simulink model "dynamic_model_dab_range_test"  (R2022b)
settings: Solver=VariableStepAuto  StartTime=0.0  StopTime=100e-2  RelTol=1e-3
undefined symbols (not defined in the file): Ion, Lithium
libraries: spsSeriesRLCBranchLib x9, spsMosfetLib x8, spsMeanLib x6, eeGeneralControl x6, spsCurrentMeasurementLib x4, spsDiscreteVariableTimeDelayLib x2, spsEdgeDetectorLib x2, spsBatteryLib x1, spsDCVoltageSourceLib x1, spsMultimeterLib x1, spsStairGeneratorLib x1, slpidlib x1
settings Model: Creator=srikr  LastModifiedBy=srikri

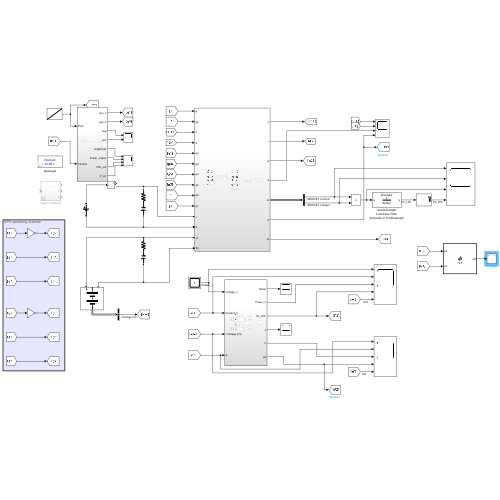
[thumbnail: Simulink's stored preview of the top-level diagram]
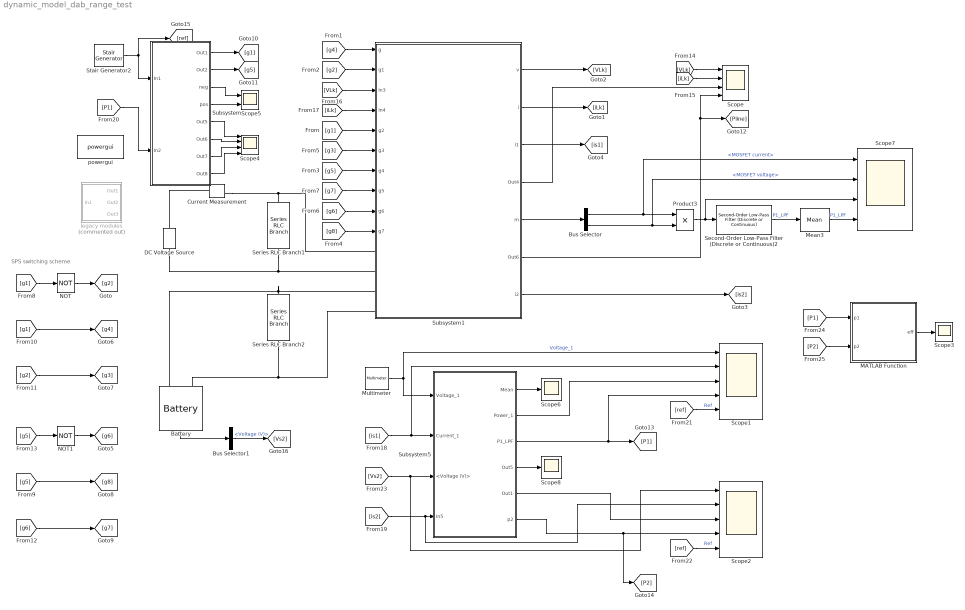
== system dynamic_model_dab_range_test ==
  note: SPS switching scheme
  Battery : spsBatteryLib/Battery  BatType=Lithium-Ion  ShowTempParam=off  ThermalPreset=no  ShowAgeParam=off  NomV=96  NomQ=150  SOC=100  Batt_Tr=30  PresetModel=on  MaxQ=150  MinV=72  FullV=111.7428  Dis_rate=65.2174  R=0.0064  Normal_OP=135.6522  expZone="[103.717      7.369565]"  current=[6.5 13 32.5]  Units=Time  Tci=20  NomT=20  T2=-30  MaxQ2=4.8  FullV2=7.1  Normal_OP2=5.655  expZone2="[6.58           1]"  Rca=0.6  ti=2000  Dp=0  Neq0=0  Tsim=1e6  Ta1=25  Qeol=5.4*0.9  Reol=0.013333*1.2  Char_age=[2.3478, 3]  Dis_age=[2.3478, 10]  N1=1500  N2=10500  N3=1000  N4=1400  Ta2=45  N5=950
  Bus Selector : BusSelector  OutputSignals=MOSFET current,MOSFET voltage
  Bus Selector1 : BusSelector  OutputSignals=Voltage (V)
  Current Measurement : spsCurrentMeasurementLib/Current Measurement  PhasorSimulation=off  OutputType=Complex  PSBequivalent=0
  DC Voltage Source : spsDCVoltageSourceLib/DC Voltage Source  Amplitude=120  Measurements=Voltage
  MATLAB Function : MATLAB Function  TreatAsAtomicUnit=on
  Mean3 : spsMeanLib/Mean  Freq=50e3  Vinit=0  Ts=0
  Multimeter : spsMultimeterLib/Multimeter  L=10  sel=4  yselected={}  Gain=1  OutputType=Complex  PlotAtSimulationStop=off  PhasorSimulation=off
  NOT : Logic  Operator=NOT  IconShape=distinctive  AllPortsSameDT=off  OutDataTypeStr=boolean
  NOT1 : Logic  Operator=NOT  IconShape=distinctive  AllPortsSameDT=off  OutDataTypeStr=boolean
  Product3 : Product
  Scope : Scope  NumInputPorts=4
  Scope1 : Scope  NumInputPorts=5
  Scope2 : Scope  NumInputPorts=5
  Scope3 : Scope
  Scope4 : Scope  NumInputPorts=4
  Scope5 : Scope  NumInputPorts=2
  Scope6 : Scope
  Scope7 : Scope  NumInputPorts=4
  Scope8 : Scope
  Second-Order Low-Pass Filter (Discrete or Continuous)2 : eeGeneralControl/Second-Order Low-Pass Filter (Discrete or Continuous)  A1=2*sqrt(2)*1e-3  A2=(1e-3)^2  init_option=Inherited from block input  x0=0  Ts=-1
      settings: LibrarySourceBlock=|
      | ee_sl_lib/General Control/Second-Order
      | Low-Pass Filter
      | (Discrete or Continuous)
  Series RLC Branch1 : spsSeriesRLCBranchLib/Series RLC Branch  LConnTagsString=__new0  RConnTagsString=__new0  BranchType=RC  Resistance=1e-9  Inductance=1e-3  SetiL0=off  InitialCurrent=0  Capacitance=1000e-6  Setx0=off  InitialVoltage=0  Measurements=None
  Series RLC Branch2 : spsSeriesRLCBranchLib/Series RLC Branch  LConnTagsString=__new0  RConnTagsString=__new0  BranchType=RC  Resistance=1e-9  Inductance=1e-3  SetiL0=off  InitialCurrent=0  Capacitance=1000e-6  Setx0=off  InitialVoltage=0  Measurements=None
  Stair Generator2 : spsStairGeneratorLib/Stair Generator  t=[0:0.025:1]*100e-2*(1-0.1)  e=([-1:0.05:1])*2.8e3  Ts=0
  Subsystem : Subsystem
  Subsystem1 : Subsystem
  Subsystem5 : Subsystem
  legacy modules : Subsystem  Commented=on
  powergui : spspowerguiLib/powergui  Priority=1  SimulationMode=Discrete  SampleTime=1e-6  frequency=60  Iterations=50  frequencyindice=0  Pbase=100e6  ErrMax=1e-4  UnitsV=kV  UnitsW=MW  buscounter=0  FunctionMessages=off  echomessages=off  EnableUseOfTLC=off  CurrentSourceSwitches=off  DisableSnubberDevices=off  DisableRonSwitches=off  DisableVfSwitches=off  DisplayEquations=off  AutomaticDiscreteSolvers=off  SolverType=Tustin/Backward Euler (TBE)  Interpol=off  ExternalGateDelay=off  methode=off  Ts=100  x0status=blocks  SPID=on  SwTol=0  HookPort=off  NonlinearTolerance=1e-4  nMaxIteration=100  ContinueOnMaxIteration=off  RestoreLinks=warning  ResistiveCurrentMeasurement=off  Frange=[0:2:500]  Ylog=off  Xlog=on  ShowGrid=off  save=off  variable=ZData  structure=0  ZoomFFT=off  StartTime=0.0  cycles=1  DisplayStyle=1  fundamental=60  FreqAxis=off  MaxFrequency=1000  frequencyindicesteady=1  RmsSteady=1  display=off
  wires:
  [VLk] -> Scope/1
  [iLk] -> Scope/2
  Multimeter/1 -> Scope1/1, Subsystem5/1(Voltage_1)  "Voltage_1"
  [is2] -> Scope2/2, Subsystem5/4(In5)
  Stair Generator2/1 -> Subsystem/1(In1), [ref]
  Bus Selector/1 -> Scope7/1, Product3/1  "<MOSFET current>"
  Bus Selector/2 -> Scope7/2, Product3/2  "<MOSFET voltage>"
  Product3/1 -> Scope7/3, Second-Order Low-Pass Filter (Discrete or Continuous)2/1
  [ref] -> Scope1/5  "Ref"
  Battery/1 -> Bus Selector1/1
  [P1] -> Subsystem/2(In2)
  Subsystem/1(Out1) -> [g1]
  Subsystem/2(Out2) -> [g5]
  Subsystem/3(neg) -> Scope5/1
  Subsystem/4(pos) -> Scope5/2
  Subsystem/5(Out5) -> Scope4/1
  Subsystem/6(Out6) -> Scope4/2
  Subsystem/7(Out7) -> Scope4/3
  Subsystem/8(Out8) -> Scope4/4
  Subsystem5/1(Mean) -> Scope6/1
  Subsystem5/2(Power_1) -> Scope1/3
  Subsystem1/6(Out6) -> [Pline], Scope/4
  [g4] -> Subsystem1/1(g)
  [g2] -> Subsystem1/2(g1)
  [VLk] -> Subsystem1/3(In3)
  [iLk] -> Subsystem1/4(In4)
  [g1] -> Subsystem1/5(g2)
  [g3] -> Subsystem1/6(g3)
  [g5] -> Subsystem1/7(g4)
  [g7] -> Subsystem1/8(g5)
  [g6] -> Subsystem1/9(g6)
  [g8] -> Subsystem1/10(g7)
  Subsystem1/1(v) -> [VLk]
  Subsystem1/2(i) -> [iLk]
  Subsystem1/3(i1) -> [is1]
  Subsystem1/4(Out4) -> Scope/3
  Subsystem1/5(m) -> Bus Selector/1
  Subsystem1/7(i2) -> [is2]
  [g1] -> NOT/1
  NOT/1 -> [g2]
  [g5] -> [g8]
  NOT1/1 -> [g6]
  [g6] -> [g7]
  [g5] -> NOT1/1
  [g2] -> [g3]
  [g1] -> [g4]
  Subsystem5/5(Out1) -> Scope2/3
  [is1] -> Scope1/2, Subsystem5/2(Current_1)
  [ref] -> Scope2/5  "Ref"
  Bus Selector1/1 -> [Vs2]  "<Voltage (V)>"
  [Vs2] -> Scope2/1, Subsystem5/3(<Voltage (V)>)
  Second-Order Low-Pass Filter (Discrete or Continuous)2/1 -> Mean3/1  "P1_LPF"
  Mean3/1 -> Scope7/4  "P1_LPF"
  Subsystem5/3(P1_LPF) -> [P1], Scope1/4
  MATLAB Function/1(eff) -> Scope3/1
  Subsystem5/4(Out5) -> Scope8/1
  Subsystem5/6(p2) -> [P2], Scope2/4
  [P1] -> MATLAB Function/1(p1)
  [P2] -> MATLAB Function/2(p2)
  connections:
  Series RLC Branch1/RConn1 -- DC Voltage Source/LConn1 -- Subsystem1/LConn2
  Series RLC Branch2/RConn1 -- Battery/LConn2 -- Subsystem1/LConn4
  Series RLC Branch2/LConn1 -- Battery/LConn1 -- Subsystem1/LConn3
  Subsystem1/LConn1 -- Current Measurement/RConn1 -- Series RLC Branch1/LConn1
  Current Measurement/LConn1 -- DC Voltage Source/RConn1

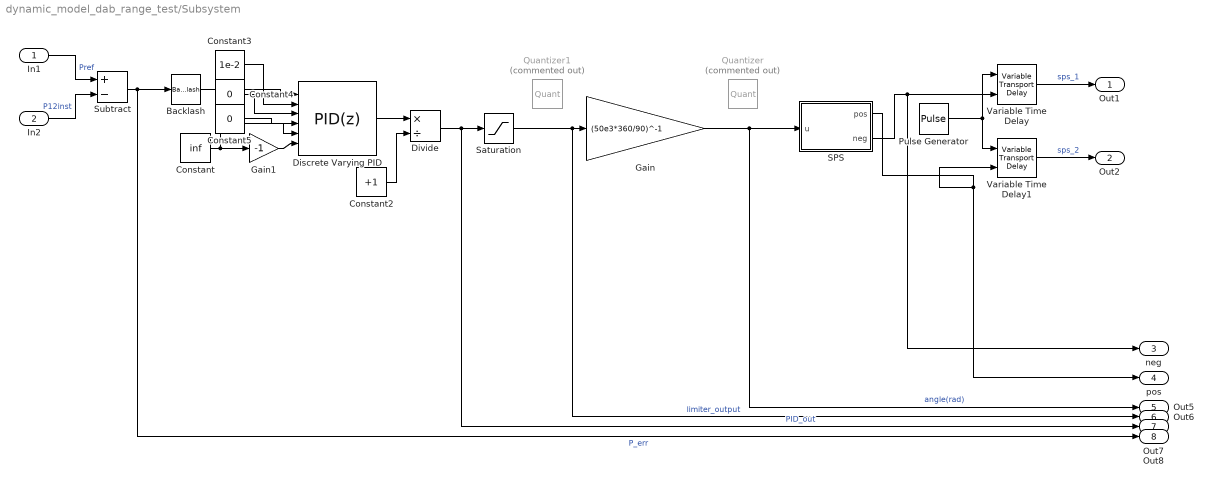
== system dynamic_model_dab_range_test/Subsystem ==
  In1 : Inport
  In2 : Inport  Port=2
  Backlash : Backlash  BacklashWidth=0
  Constant : Constant  Value=inf
  Constant2 : Constant  Value=+1
  Constant3 : Constant  Value=1e-2
  Constant4 : Constant  Value=0
  Constant5 : Constant  Value=0
  Discrete Varying PID : slpidlib/PID Controller  Controller=PID  Form=Parallel  TimeDomain=Discrete-time  UseExternalTs=off  SampleTime=-1  IntegratorMethod=Forward Euler  FilterMethod=Forward Euler  ControllerParametersSource=external  P=1  I=1  UseKiTs=off  D=0  N=100  UseFilter=off  TunerSelectOption=Transfer Function Based (PID Tuner App)  InitialConditionSource=internal  InitialConditionForIntegrator=0  InitialConditionForFilter=0  DifferentiatorICPrevScaledInput=0  ExternalReset=none  TrackingMode=off  Kt=1  LimitOutput=on  SatLimitsSource=external  UpperSaturationLimit=inf  LowerSaturationLimit=-inf  LinearizeAsGain=on  AntiWindupMode=none  Kb=1  LimitIntegrator=off  UpperIntegratorSaturationLimit=inf  LowerIntegratorSaturationLimit=-inf  POutMin=[]  POutMax=[]  IOutMin=[]  IOutMax=[]  DOutMin=[]  DOutMax=[]  NOutMin=[]  NOutMax=[]  SumOutMin=[]  SumOutMax=[]  SaturationOutMin=[]  SaturationOutMax=[]  PParamMin=[]  PParamMax=[]  IParamMin=[]  IParamMax=[]  DParamMin=[]  DParamMax=[]  NParamMin=[]  NParamMax=[]  KbParamMin=[]  KbParamMax=[]  KtParamMin=[]  KtParamMax=[]  KbOutMin=[]  KbOutMax=[]  KtOutMin=[]  KtOutMax=[]  IntegratorOutMin=[]  IntegratorOutMax=[]  FilterOutMin=[]  FilterOutMax=[]  SumI1OutMin=[]  SumI1OutMax=[]  SumI2OutMin=[]  SumI2OutMax=[]  SumI3OutMin=[]  SumI3OutMax=[]  SumI4OutMin=[]  SumI4OutMax=[]  SumDOutMin=[]  SumDOutMax=[]  DifferentiatorOutMin=[]  DifferentiatorOutMax=[]  FilterDiffOutCoefMin=[]  FilterDiffOutCoefMax=[]  ReciprocalOutMin=[]  ReciprocalOutMax=[]  SumDenOutMin=[]  SumDenOutMax=[]  SumNumOutMin=[]  SumNumOutMax=[]  DivideOutMin=[]  DivideOutMax=[]  UdiffTsProdOutMin=[]  UdiffTsProdOutMax=[]  NTsProdOutMin=[]  NTsProdOutMax=[]  UintegralTsProdOutMin=[]  UintegralTsProdOutMax=[]  UngainTsProdOutMin=[]  UngainTsProdOutMax=[]  ClampingZeroOutDataTypeStr=Inherit: Inherit via back propagation  ClampingZeroOutMin=[]  ClampingZeroOutMax=[]  FilterDenConstantOutDataTypeStr=Inherit: Inherit via back propagation  FilterDenConstantOutMin=[]  FilterDenConstantOutMax=[]  PCopyOutDataTypeStr=Inherit: Inherit via back propagation  PCopyOutMin=[]  PCopyOutMax=[]  NCopyOutDataTypeStr=Inherit: Inherit via back propagation  NCopyOutMin=[]  NCopyOutMax=[]  IntegratorContinuousStateAttributes=''  IntegratorStateMustResolveToSignalObject=off  IntegratorRTWStateStorageClass=Auto  FilterContinuousStateAttributes=''  FilterStateMustResolveToSignalObject=off  FilterRTWStateStorageClass=Auto  ParallelPVariant=ExternalParameters  IdealPVariant=Disabled  IVariant=ExternalParameters  DVariant=ExternalParameters  IntegratorVariant=Discrete  SatVariant=External  AWVariant=Passthrough  PCopyVariant=Disabled  TRVariant=Disabled  FdbkBlocksVariant=Forward  IdealPFdbkVariant=Disabled  SatFdbkVariant=Disabled  DerivativeFilterVariant=Differentiator  NVariant=Passthrough  NCopyVariant=Disabled_SignalSpec  FilterICVariant=InternalICsDifferentiator  IntegratorICVariant=InternalICs  ExternalResetVariant=Disabled  TRSumVariant=Passthrough  SumFdbkVariant=Disabled  SumVariant=Sum_PID  TsampFilterVariant=InternalTs  TsampNgainVariant=Passthrough  TsampIntegralVariant=Passthrough  ExternalSaturationOutDataTypeStr=Inherit: Same as second input
      settings: LibrarySourceBlock=cstblocks/Linear Parameter Varying/Discrete Varying PID
  Divide : Product  Inputs=*/
  Gain : Gain  Gain=(50e3*360/90)^-1
  Gain1 : Gain  Gain=-1
  Pulse Generator : DiscretePulseGenerator  PulseType=Time based  Period=1/50e3  PulseWidth=50
  Quantizer : Quantizer  Commented=on  QuantizationInterval=1e-5
  Quantizer1 : Quantizer  Commented=on  QuantizationInterval=1e-2
  SPS : MATLAB Function  TreatAsAtomicUnit=on
  Saturation : Saturate  UpperLimit=1  LowerLimit=-1
  Subtract : Sum  Inputs=+-
  Variable Time Delay : VariableTransportDelay  MaximumDelay=10
  Variable Time Delay1 : VariableTransportDelay  MaximumDelay=10
  Out1 : Outport
  Out2 : Outport  Port=2
  neg : Outport  Port=3
  pos : Outport  Port=4
  Out5 : Outport  Port=5
  Out6 : Outport  Port=6
  Out7 : Outport  Port=7
  Out8 : Outport  Port=8
  wires:
  Backlash/1 -> Discrete Varying PID/1
  Constant2/1 -> Divide/2
  Constant4/1 -> Discrete Varying PID/3
  In1/1 -> Subtract/1  "Pref"
  Variable Time Delay/1 -> Out1/1  "sps_1"
  Saturation/1 -> Out6/1, Gain/1  "limiter_output"
  SPS/1(pos) -> pos/1, Variable Time Delay1/2
  SPS/2(neg) -> neg/1, Variable Time Delay/2
  Variable Time Delay1/1 -> Out2/1  "sps_2"
  In2/1 -> Subtract/2  "P12inst"
  Constant/1 -> Discrete Varying PID/5, Gain1/1
  Constant5/1 -> Discrete Varying PID/4
  Pulse Generator/1 -> Variable Time Delay1/1, Variable Time Delay/1
  Constant3/1 -> Discrete Varying PID/2
  Divide/1 -> Out7/1, Saturation/1  "PID_out"
  Discrete Varying PID/1 -> Divide/1
  Subtract/1 -> Out8/1, Backlash/1  "P_err"
  Gain1/1 -> Discrete Varying PID/6
  Gain/1 -> Out5/1, SPS/1(u)  "angle(rad)"

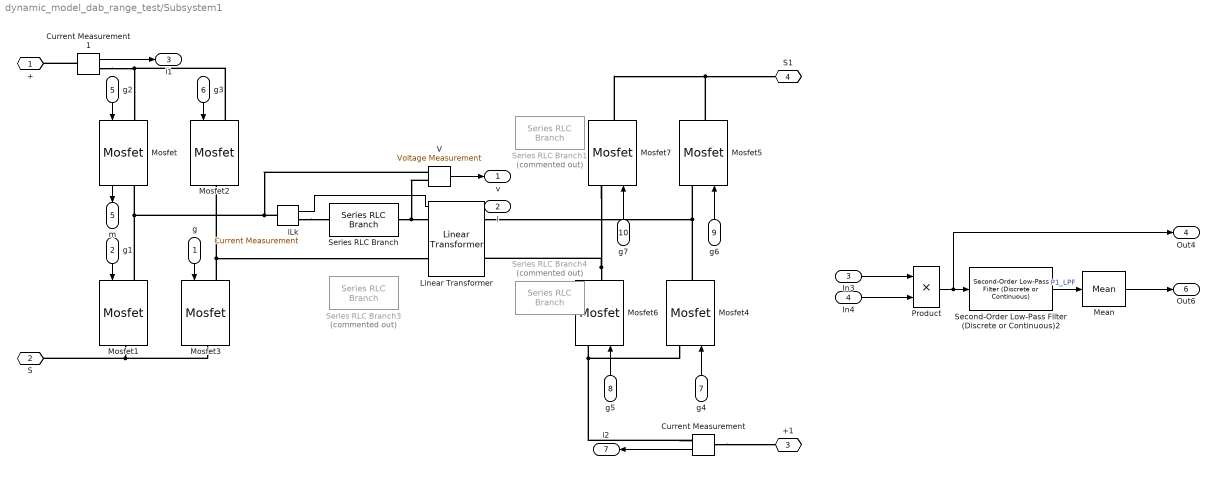
== system dynamic_model_dab_range_test/Subsystem1 ==
  g : Inport
  g1 : Inport  Port=2
  In3 : Inport  Port=3
  In4 : Inport  Port=4
  g2 : Inport  Port=5
  g3 : Inport  Port=6
  g4 : Inport  Port=7
  g5 : Inport  Port=8
  g6 : Inport  Port=9
  g7 : Inport  Port=10
  Current Measurement : spsCurrentMeasurementLib/Current Measurement  PhasorSimulation=off  OutputType=Complex  PSBequivalent=0
  Current Measurement1 : spsCurrentMeasurementLib/Current Measurement  PhasorSimulation=off  OutputType=Complex  PSBequivalent=0
  Linear Transformer : spsLinearTransformerLib/Linear Transformer  UNITS=SI  NominalPower=[ 3.5e3 50e3 ]  winding1=[120 0 0]  winding2=[96 0 0]  ThreeWindings=off  winding3=[3.15e+05 0.7938 0.084225]  RmLm=[10e6 2e-3]  Measurements=All voltages and currents  DataType=on
  Mean : spsMeanLib/Mean  Freq=50e3  Vinit=0  Ts=0
  Mosfet : spsMosfetLib/Mosfet  Ron=0.1  Lon=0  Rd=0.01  Vfd=0  IC=0  Rs=1e6  Cs=inf  Measurements=on
  Mosfet1 : spsMosfetLib/Mosfet  Ron=0.1  Lon=0  Rd=0.01  Vfd=0  IC=0  Rs=inf  Cs=inf  Measurements=off
  Mosfet{2..7} (6 alike) : spsMosfetLib/Mosfet  Ron=0.1  Lon=0  Rd=0.01  Vfd=0  IC=0  Rs=1e6  Cs=inf  Measurements=off
  Product : Product
  Second-Order Low-Pass Filter (Discrete or Continuous)2 : eeGeneralControl/Second-Order Low-Pass Filter (Discrete or Continuous)  A1=2*sqrt(2)*1e-3  A2=(1e-3)^2  init_option=Inherited from block input  x0=0  Ts=-1
      settings: LibrarySourceBlock=|
      | ee_sl_lib/General Control/Second-Order
      | Low-Pass Filter
      | (Discrete or Continuous)
  Series RLC Branch : spsSeriesRLCBranchLib/Series RLC Branch  LConnTagsString=__new0  RConnTagsString=__new0  BranchType=L  Resistance=1  Inductance=14e-6  SetiL0=off  InitialCurrent=0  Capacitance=1e-6  Setx0=off  InitialVoltage=0  Measurements=Branch voltage and current
  Series RLC Branch1 : spsSeriesRLCBranchLib/Series RLC Branch  Commented=on  LConnTagsString=__new0  RConnTagsString=__new0  BranchType=L  Resistance=1  Inductance=80e-6  SetiL0=off  InitialCurrent=0  Capacitance=1e-6  Setx0=off  InitialVoltage=0  Measurements=Branch voltage and current
  Series RLC Branch3 : spsSeriesRLCBranchLib/Series RLC Branch  Commented=on  LConnTagsString=__new0  RConnTagsString=__new0  BranchType=C  Resistance=1  Inductance=15e-6  SetiL0=off  InitialCurrent=0  Capacitance=0.127e-6  Setx0=off  InitialVoltage=0  Measurements=Branch voltage and current
  Series RLC Branch4 : spsSeriesRLCBranchLib/Series RLC Branch  Commented=on  LConnTagsString=__new0  RConnTagsString=__new0  BranchType=C  Resistance=1  Inductance=15e-6  SetiL0=off  InitialCurrent=0  Capacitance=0.127e-6  Setx0=off  InitialVoltage=0  Measurements=Branch voltage and current
  V : spsVoltageMeasurementLib/Voltage Measurement  PhasorSimulation=off  OutputType=Complex  PSBequivalent=0
  iLk : spsCurrentMeasurementLib/Current Measurement  PhasorSimulation=off  OutputType=Complex  PSBequivalent=0
  + : PMIOPort  Side=Left
  S : PMIOPort  Port=2  Side=Left
  +1 : PMIOPort  Port=3  Side=Left
  S1 : PMIOPort  Port=4  Side=Left
  v : Outport
  i : Outport  Port=2
  i1 : Outport  Port=3
  Out4 : Outport  Port=4
  m : Outport  Port=5
  Out6 : Outport  Port=6
  i2 : Outport  Port=7
  wires:
  V/1 -> v/1
  g5/1 -> Mosfet6/1
  In3/1 -> Product/1
  g6/1 -> Mosfet5/1
  In4/1 -> Product/2
  Mosfet/1 -> m/1
  g2/1 -> Mosfet/1
  g4/1 -> Mosfet4/1
  iLk/1 -> i/1
  Current Measurement1/1 -> i1/1
  Current Measurement/1 -> i2/1
  g1/1 -> Mosfet1/1
  g/1 -> Mosfet3/1
  Mean/1 -> Out6/1
  g3/1 -> Mosfet2/1
  g7/1 -> Mosfet7/1
  Product/1 -> Out4/1, Second-Order Low-Pass Filter (Discrete or Continuous)2/1
  Second-Order Low-Pass Filter (Discrete or Continuous)2/1 -> Mean/1  "P1_LPF"
  connections:
  Current Measurement1/RConn1 -- Mosfet/LConn1 -- Mosfet2/LConn1
  Series RLC Branch/RConn1 -- V/LConn2 -- Linear Transformer/LConn1
  Current Measurement/LConn1 -- +1/RConn1
  Current Measurement/RConn1 -- Mosfet4/LConn1 -- Mosfet6/LConn1
  Current Measurement1/LConn1 -- +/RConn1
  Mosfet3/RConn1 -- S/RConn1 -- Mosfet1/RConn1
  iLk/LConn1 -- V/LConn1 -- Mosfet/RConn1 -- Mosfet1/LConn1
  iLk/RConn1 -- Series RLC Branch/LConn1
  Mosfet7/RConn1 -- Mosfet5/RConn1 -- S1/RConn1
  Mosfet3/LConn1 -- Linear Transformer/LConn2 -- Mosfet2/RConn1
  Mosfet4/RConn1 -- Mosfet5/LConn1 -- Linear Transformer/RConn1
  Mosfet6/RConn1 -- Linear Transformer/RConn2 -- Mosfet7/LConn1

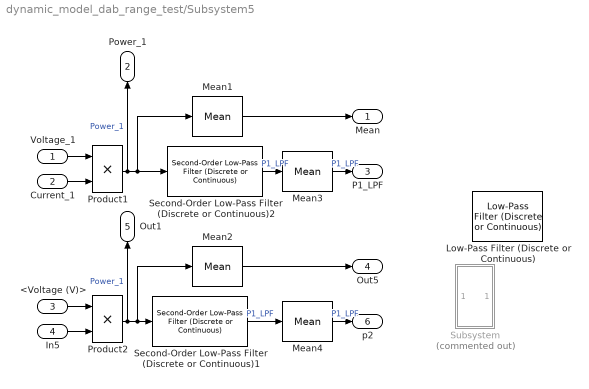
== system dynamic_model_dab_range_test/Subsystem5 ==
  Voltage_1 : Inport
  Current_1 : Inport  Port=2
  <Voltage (V)> : Inport  Port=3
  In5 : Inport  Port=4
  Low-Pass Filter (Discrete or Continuous) : eeGeneralControl/Low-Pass Filter (Discrete or Continuous)  K=1  T=1e-3  B=inf  A=-inf  init_option=Specify as parameter  x0=0  Ts=-1
  Mean{1..4} (4 alike) : spsMeanLib/Mean  Freq=50e3  Vinit=0  Ts=0
  Product1 : Product
  Product2 : Product
  Second-Order Low-Pass Filter (Discrete or Continuous)1 : eeGeneralControl/Second-Order Low-Pass Filter (Discrete or Continuous)  A1=1e-3  A2=1e-6  init_option=Inherited from block input  x0=0  Ts=-1
      settings: LibrarySourceBlock=|
      | ee_sl_lib/General Control/Second-Order
      | Low-Pass Filter
      | (Discrete or Continuous)
  Second-Order Low-Pass Filter (Discrete or Continuous)2 : eeGeneralControl/Second-Order Low-Pass Filter (Discrete or Continuous)  A1=2*sqrt(2)*1e-3  A2=(1e-3)^2  init_option=Inherited from block input  x0=0  Ts=-1
      settings: LibrarySourceBlock=|
      | ee_sl_lib/General Control/Second-Order
      | Low-Pass Filter
      | (Discrete or Continuous)
  Subsystem : Subsystem  Commented=on
  Mean : Outport
  Power_1 : Outport  Port=2
  P1_LPF : Outport  Port=3
  Out5 : Outport  Port=4
  Out1 : Outport  Port=5
  p2 : Outport  Port=6
  wires:
  Current_1/1 -> Product1/2
  Mean1/1 -> Mean/1
  Product1/1 -> Mean1/1, Second-Order Low-Pass Filter (Discrete or Continuous)2/1, Power_1/1  "Power_1"
  <Voltage (V)>/1 -> Product2/1
  Voltage_1/1 -> Product1/1
  In5/1 -> Product2/2
  Mean2/1 -> Out5/1
  Mean3/1 -> P1_LPF/1  "P1_LPF"
  Second-Order Low-Pass Filter (Discrete or Continuous)1/1 -> Mean4/1  "P1_LPF"
  Product2/1 -> Mean2/1, Second-Order Low-Pass Filter (Discrete or Continuous)1/1, Out1/1  "Power_1"
  Mean4/1 -> p2/1  "P1_LPF"
  Second-Order Low-Pass Filter (Discrete or Continuous)2/1 -> Mean3/1  "P1_LPF"

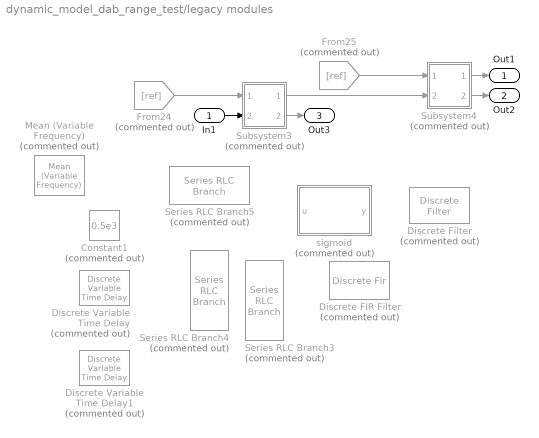
== system dynamic_model_dab_range_test/legacy modules ==
  In1 : Inport
  Constant1 : Constant  Commented=on  Value=0.5e3
  Discrete FIR Filter : DiscreteFir  Commented=on
  Discrete Filter : DiscreteFilter  Commented=on
  Discrete Variable Time Delay : spsDiscreteVariableTimeDelayLib/Discrete Variable Time Delay  Commented=on  MaxDelay=1  InitialValue=0  Ts=1e-4  DFT=on
      settings: LibrarySourceBlock=|
      | sps_lib/Control/Discrete Variable
      | Time Delay
  Discrete Variable Time Delay1 : spsDiscreteVariableTimeDelayLib/Discrete Variable Time Delay  Commented=on  MaxDelay=1  InitialValue=0  Ts=1e-4  DFT=on
      settings: LibrarySourceBlock=|
      | sps_lib/Control/Discrete Variable
      | Time Delay
  From24 : From  Commented=on  GotoTag=ref
  From25 : From  Commented=on  GotoTag=ref
  Mean (Variable Frequency) : spsMeanVariableFrequencyLib/Mean (Variable Frequency)  Commented=on  Finit=60  Fmin=45  Vinit=0  Ts=0
      settings: LibrarySourceBlock=|
      | sps_lib/Sensors and Measurements/Mean
      | (Variable Frequency)
  Series RLC Branch3 : spsSeriesRLCBranchLib/Series RLC Branch  Commented=on  LConnTagsString=__new0  RConnTagsString=__new0  BranchType=L  Resistance=1  Inductance=1e-6/(1.25^2)  SetiL0=off  InitialCurrent=0  Capacitance=1e-6  Setx0=off  InitialVoltage=0  Measurements=Branch voltage and current
  Series RLC Branch4 : spsSeriesRLCBranchLib/Series RLC Branch  Commented=on  LConnTagsString=__new0  RConnTagsString=__new0  BranchType=C  Resistance=1  Inductance=14e-6  SetiL0=off  InitialCurrent=0  Capacitance=10e-6*(1.25^2)  Setx0=off  InitialVoltage=0  Measurements=Branch voltage and current
  Series RLC Branch5 : spsSeriesRLCBranchLib/Series RLC Branch  Commented=on  LConnTagsString=__new0  RConnTagsString=__new0  BranchType=C  Resistance=1  Inductance=14e-6  SetiL0=off  InitialCurrent=0  Capacitance=10e-6  Setx0=off  InitialVoltage=0  Measurements=Branch voltage and current
  Subsystem3 : Subsystem  Commented=on
  Subsystem4 : Subsystem  Commented=on
  sigmoid : MATLAB Function  Commented=on  TreatAsAtomicUnit=on
  Out1 : Outport
  Out2 : Outport  Port=2
  Out3 : Outport  Port=3
  wires:
  Subsystem3/1(Out1) -> Subsystem4/2(In2)
  From25/1 -> Subsystem4/1(In1)
  From24/1 -> Subsystem3/1(In1)
  In1/1 -> Subsystem3/2(In2)
  Subsystem4/2(Out2) -> Out2/1
  Subsystem4/1(Out1) -> Out1/1
  Subsystem3/2(Out2) -> Out3/1

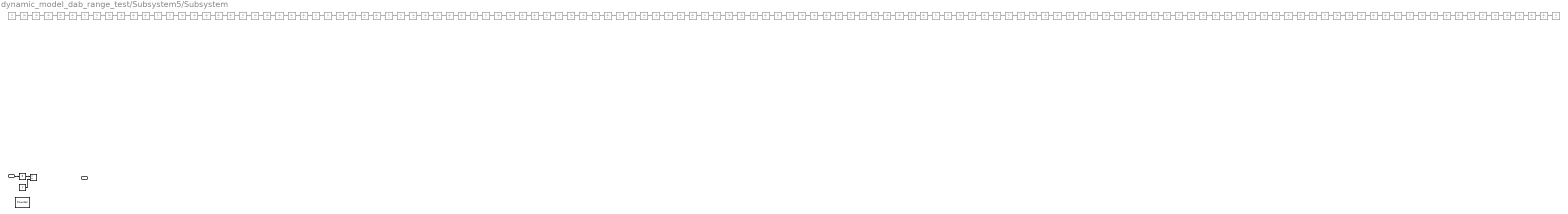
== system dynamic_model_dab_range_test/Subsystem5/Subsystem ==
  In1 : Inport
  Constant : Constant
  Counter : eeGeneralControl/Counter  CarrCount=Up  Range=[0 1]  Tper=0.001  Tdelay=0  Ts=0.0001
      settings: LibrarySourceBlock=ee_sl_lib/General Control/Counter
  Divide : Product  Inputs=*/
  Sum of Elements : Sum  Inputs=+  AccumDataTypeStr=int16  SaturateOnIntegerOverflow=on
  Unit Delay{,1..127} (128 alike) : UnitDelay  Commented=on  SampleTime=-1  HasFrameUpgradeWarning=on
  Out1 : Outport
  wires:
  In1/1 -> Sum of Elements/1
  Unit Delay65/1 -> Unit Delay120/1
  Unit Delay126/1 -> Unit Delay127/1
  Unit Delay2/1 -> Unit Delay3/1
  Unit Delay64/1 -> Unit Delay65/1
  Unit Delay125/1 -> Unit Delay98/1
  Unit Delay/1 -> Unit Delay1/1
  Unit Delay82/1 -> Unit Delay72/1
  Unit Delay75/1 -> Unit Delay88/1
  Unit Delay88/1 -> Unit Delay89/1
  Unit Delay72/1 -> Unit Delay73/1
  Unit Delay86/1 -> Unit Delay83/1
  Unit Delay40/1 -> Unit Delay41/1
  Unit Delay17/1 -> Unit Delay28/1
  Unit Delay69/1 -> Unit Delay81/1
  Unit Delay116/1 -> Unit Delay117/1
  Unit Delay87/1 -> Unit Delay64/1
  Unit Delay10/1 -> Unit Delay11/1
  Unit Delay96/1 -> Unit Delay97/1
  Unit Delay78/1 -> Unit Delay103/1
  Unit Delay115/1 -> Unit Delay90/1
  Unit Delay46/1 -> Unit Delay76/1
  Unit Delay77/1 -> Unit Delay78/1
  Unit Delay90/1 -> Unit Delay91/1
  Unit Delay98/1 -> Unit Delay109/1
  Unit Delay26/1 -> Unit Delay27/1
  Unit Delay100/1 -> Unit Delay113/1
  Unit Delay68/1 -> Unit Delay69/1
  Unit Delay120/1 -> Unit Delay125/1
  Unit Delay12/1 -> Unit Delay13/1
  Unit Delay112/1 -> Unit Delay101/1
  Unit Delay50/1 -> Unit Delay40/1
  Unit Delay103/1 -> Unit Delay115/1
  Unit Delay80/1 -> Unit Delay77/1
  Unit Delay124/1 -> Unit Delay96/1
  Unit Delay38/1 -> Unit Delay39/1
  Unit Delay84/1 -> Unit Delay74/1
  Unit Delay73/1 -> Unit Delay85/1
  Unit Delay56/1 -> Unit Delay57/1
  Unit Delay118/1 -> Unit Delay119/1
  Unit Delay89/1 -> Unit Delay79/1
  Unit Delay44/1 -> Unit Delay55/1
  Unit Delay94/1 -> Unit Delay95/1
  Unit Delay43/1 -> Unit Delay56/1
  Unit Delay81/1 -> Unit Delay82/1
  Unit Delay79/1 -> Unit Delay80/1
  Unit Delay58/1 -> Unit Delay59/1
  Unit Delay24/1 -> Unit Delay25/1
  Unit Delay85/1 -> Unit Delay86/1
  Unit Delay97/1 -> Unit Delay94/1
  Unit Delay104/1 -> Unit Delay105/1
  Unit Delay71/1 -> Unit Delay68/1
  Unit Delay127/1 -> Unit Delay70/1
  Unit Delay76/1 -> Unit Delay87/1
  Unit Delay7/1 -> Unit Delay4/1
  Unit Delay108/1 -> Unit Delay110/1
  Unit Delay110/1 -> Unit Delay99/1
  Unit Delay107/1 -> Unit Delay104/1
  Unit Delay117/1 -> Unit Delay106/1
  Unit Delay54/1 -> Unit Delay51/1
  Unit Delay61/1 -> Unit Delay58/1
  Unit Delay122/1 -> Unit Delay118/1
  Unit Delay93/1 -> Unit Delay123/1
  Unit Delay59/1 -> Unit Delay34/1
  Unit Delay51/1 -> Unit Delay52/1
  Unit Delay114/1 -> Unit Delay111/1
  Unit Delay95/1 -> Unit Delay108/1
  Unit Delay83/1 -> Unit Delay84/1
  Unit Delay106/1 -> Unit Delay107/1
  Unit Delay13/1 -> Unit Delay24/1
  Unit Delay113/1 -> Unit Delay114/1
  Unit Delay91/1 -> Unit Delay121/1
  Unit Delay25/1 -> Unit Delay16/1
  Unit Delay121/1 -> Unit Delay122/1
  Unit Delay66/1 -> Unit Delay67/1
  Unit Delay29/1 -> Unit Delay26/1
  Unit Delay101/1 -> Unit Delay102/1
  Unit Delay111/1 -> Unit Delay112/1
  Unit Delay30/1 -> Unit Delay31/1
  Unit Delay70/1 -> Unit Delay71/1
  Unit Delay119/1 -> Unit Delay92/1
  Unit Delay18/1 -> Unit Delay19/1
  Unit Delay67/1 -> Unit Delay126/1
  Unit Delay74/1 -> Unit Delay75/1
  Unit Delay28/1 -> Unit Delay29/1
  Unit Delay102/1 -> Unit Delay116/1
  Unit Delay6/1 -> Unit Delay7/1
  Unit Delay31/1 -> Unit Delay22/1
  Unit Delay63/1 -> Unit Delay38/1
  Unit Delay16/1 -> Unit Delay17/1
  Unit Delay19/1 -> Unit Delay30/1
  Unit Delay22/1 -> Unit Delay23/1
  Unit Delay20/1 -> Unit Delay21/1
  Unit Delay62/1 -> Unit Delay63/1
  Unit Delay32/1 -> Unit Delay33/1
  Unit Delay39/1 -> Unit Delay36/1
  Unit Delay35/1 -> Unit Delay62/1
  Unit Delay37/1 -> Unit Delay49/1
  Unit Delay33/1 -> Unit Delay60/1
  Unit Delay3/1 -> Unit Delay/1
  Unit Delay21/1 -> Unit Delay44/1
  Unit Delay47/1 -> Unit Delay48/1
  Unit Delay42/1 -> Unit Delay43/1
  Unit Delay60/1 -> Unit Delay61/1
  Unit Delay41/1 -> Unit Delay53/1
  Unit Delay23/1 -> Unit Delay20/1
  Unit Delay55/1 -> Unit Delay32/1
  Unit Delay34/1 -> Unit Delay35/1
  Unit Delay11/1 -> Unit Delay8/1
  Unit Delay15/1 -> Unit Delay12/1
  Unit Delay14/1 -> Unit Delay15/1
  Unit Delay53/1 -> Unit Delay54/1
  Unit Delay99/1 -> Unit Delay100/1
  Unit Delay49/1 -> Unit Delay50/1
  Unit Delay45/1 -> Unit Delay46/1
  Unit Delay9/1 -> Unit Delay14/1
  Unit Delay36/1 -> Unit Delay37/1
  Unit Delay123/1 -> Unit Delay124/1
  Unit Delay109/1 -> Unit Delay66/1
  Unit Delay92/1 -> Unit Delay93/1
  Unit Delay5/1 -> Unit Delay10/1
  Unit Delay48/1 -> Unit Delay45/1
  Unit Delay57/1 -> Unit Delay47/1
  Unit Delay52/1 -> Unit Delay42/1
  Unit Delay27/1 -> Unit Delay18/1
  Unit Delay4/1 -> Unit Delay5/1
  Unit Delay8/1 -> Unit Delay9/1
  Unit Delay1/1 -> Unit Delay6/1
  Sum of Elements/1 -> Divide/1
  Constant/1 -> Divide/2

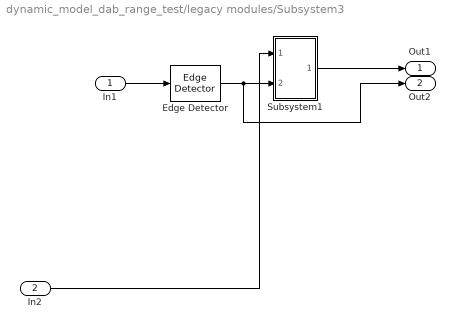
== system dynamic_model_dab_range_test/legacy modules/Subsystem3 ==
  In1 : Inport
  In2 : Inport  Port=2
  Edge Detector : spsEdgeDetectorLib/Edge Detector  model=Either  ic=0  Ts=0
      settings: LibrarySourceBlock=sps_lib/Control/Edge Detector
  Subsystem1 : Subsystem
  Out1 : Outport
  Out2 : Outport  Port=2
  wires:
  Edge Detector/1 -> Out2/1, Subsystem1/2(Input)
  Subsystem1/1(Out1) -> Out1/1
  In1/1 -> Edge Detector/1
  In2/1 -> Subsystem1/1(In1)

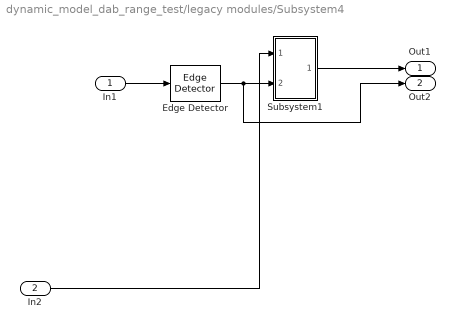
== system dynamic_model_dab_range_test/legacy modules/Subsystem4 ==
  In1 : Inport
  In2 : Inport  Port=2
  Edge Detector : spsEdgeDetectorLib/Edge Detector  model=Either  ic=0  Ts=0
      settings: LibrarySourceBlock=sps_lib/Control/Edge Detector
  Subsystem1 : Subsystem
  Out1 : Outport
  Out2 : Outport  Port=2
  wires:
  Edge Detector/1 -> Out2/1, Subsystem1/2(Input)
  Subsystem1/1(Out1) -> Out1/1
  In1/1 -> Edge Detector/1
  In2/1 -> Subsystem1/1(In1)

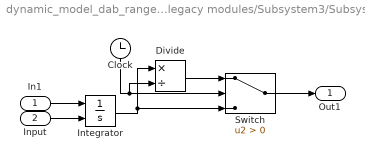
== system dynamic_model_dab_range_test/legacy modules/Subsystem3/Subsystem1 ==
  In1 : Inport
  Input : Inport  Port=2
  Clock : Clock
  Divide : Product  Inputs=*/
  Integrator : Integrator  ExternalReset=rising  LimitOutput=on  IgnoreLimit=on
  Switch : Switch  Criteria=u2 > Threshold  SaturateOnIntegerOverflow=off  InputSameDT=off
  Out1 : Outport
  wires:
  Divide/1 -> Switch/1
  Integrator/1 -> Switch/3, Divide/1
  Clock/1 -> Switch/2, Divide/2
  In1/1 -> Integrator/1
  Switch/1 -> Out1/1
  Input/1 -> Integrator/2

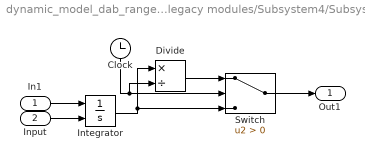
== system dynamic_model_dab_range_test/legacy modules/Subsystem4/Subsystem1 ==
  In1 : Inport
  Input : Inport  Port=2
  Clock : Clock
  Divide : Product  Inputs=*/
  Integrator : Integrator  ExternalReset=rising  LimitOutput=on  IgnoreLimit=on
  Switch : Switch  Criteria=u2 > Threshold  SaturateOnIntegerOverflow=off  InputSameDT=off
  Out1 : Outport
  wires:
  Divide/1 -> Switch/1
  Integrator/1 -> Switch/3, Divide/1
  Clock/1 -> Switch/2, Divide/2
  In1/1 -> Integrator/1
  Switch/1 -> Out1/1
  Input/1 -> Integrator/2

== matlab function dynamic_model_dab_range_test/legacy modules/sigmoid ==
  data: u input; y output
function y = fcn(u)

y = 1/(1 + exp(-u));

== matlab function dynamic_model_dab_range_test/MATLAB Function ==
  data: p1 input; eff output; p2 input
function eff = fcn(p1,p2)

eff = 100*(1-abs(p1+p2)/max(abs(p1),abs(p2)));

== matlab function dynamic_model_dab_range_test/Subsystem/SPS ==
  data: u input; pos output; neg output
function [pos,neg] = fcn(u)

if u>=0
    pos = abs(u);
    neg = 0;
else
    neg = abs(u);
    pos = 0;
end
